simulink model "BoostQuadSimu"  (R2021b)
settings: Solver=VariableStepAuto  StartTime=0.0  StopTime=Tsim  RelTol=1e-3
undefined symbols (not defined in the file): BoostQ, Dc, PRBS_Amp, PRBS_N, PRBS_Ts, Ramp_Max, Tsim
libraries: fl_lib x14, nesl_utility x11, ee_lib x5, spsPWMGeneratorDCDCLib x1
settings Model: Creator=marcus  LastModifiedBy=Gabri
settings SolverCC: AlgebraicLoopSolver=TrustRegion
settings DataIOCC: ReturnWorkspaceOutputs=off
settings DebuggingCC: SFMachineParentedDataDiag=warning  ArithmeticOperatorsInVariantConditions=warning
settings SFSimCC: SimUseLocalCustomCode=off  CustomCodeUndefinedFunction=UseInterfaceOnly
settings RTWCC: RTWUseLocalCustomCode=off

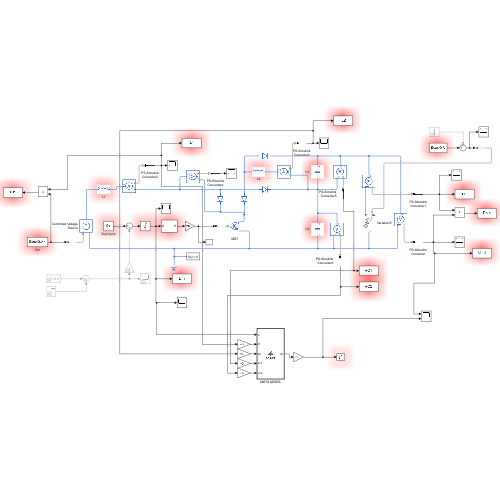
[thumbnail: Simulink's stored preview of the top-level diagram]
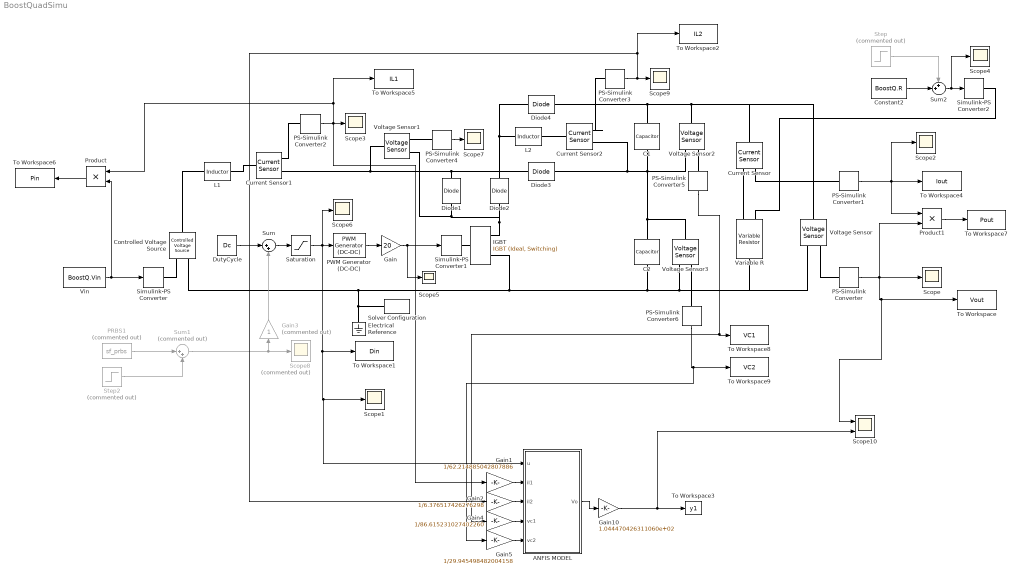
== system BoostQuadSimu ==
  ANFIS MODEL : MATLAB Function  TreatAsAtomicUnit=on
  C1 : fl_lib/Electrical/Electrical Elements/Capacitor  c=BoostQ.C1 F  r=BoostQ.rC1 Ohm  g=0 1/Ohm  i_specify=off  i_priority=None  i=0 A  i_nominal_specify=off  i_nominal_unit=A  i_nominal_value=1  v_specify=on  v_priority=High  v=vc1 V  v_nominal_specify=off  v_nominal_unit=V  v_nominal_value=1  vc_specify=off  vc_priority=None  vc=BoostQ.Vin/2 V  vc_nominal_specify=off  vc_nominal_unit=V  vc_nominal_value=1
  C2 : fl_lib/Electrical/Electrical Elements/Capacitor  c=BoostQ.C2 F  r=BoostQ.rC2 Ohm  g=0 1/Ohm  i_specify=off  i_priority=None  i=0 A  i_nominal_specify=off  i_nominal_unit=A  i_nominal_value=1  v_specify=on  v_priority=High  v=vc2 V  v_nominal_specify=off  v_nominal_unit=V  v_nominal_value=1  vc_specify=off  vc_priority=Low  vc=BoostQ.Vin V  vc_nominal_specify=off  vc_nominal_unit=V  vc_nominal_value=1
  Constant2 : Constant  Value=BoostQ.R
  Controlled Voltage Source : fl_lib/Electrical/Electrical Sources/Controlled Voltage Source
  Current Sensor : fl_lib/Electrical/Electrical Sensors/Current Sensor
  Current Sensor1 : fl_lib/Electrical/Electrical Sensors/Current Sensor
  Current Sensor2 : fl_lib/Electrical/Electrical Sensors/Current Sensor
  Diode{1..4} (4 alike) : ee_lib/Semiconductors & Converters/Diode  ModelType=ee.enum.diode.modelType.pwl  TableType=ee.enum.diode.tableType.IfMat  IfMat=[.07, .12, .19, 1.75, 4.24, 7.32, 11.2; .16, .3, .72, 2.14, 5.02, 8.35, 13.12] A  VfMat=[.9, 1.15, 1.25, 1.5, 1.75, 2.17, 2.6, 2.85; .58, .68, .75, 1.1, 1.38, 1.77, 2.27, 2.7] V  TjVec=[25, 125] degC  VfVec=[.5, .7, .9, 1.3, 1.7, 2.1, 2.5] V  IfVec=[.1, .2, .5, 1, 2, 4, 7, 10] A  Vf=0.01 V  Ron=0.01 Ohm  Goff=1e-5 1/Ohm  prmExp=ee.enum.diode.expParam.useTwo  I12=[.0137, .545] A  V12=[.6, .7] V  RS=0 Ohm  Tmeas=25 degC  IS=1e-12 A  ec=1  I1=0.0137 A  V1=0.6 V  N_series=1  N_parallel=1  Rz=0.3 Ohm  BV=inf V  C_param=ee.enum.diode.capParam.fixed  CJ=0 pF  CJ0=5 pF  Vvec=[.1, 10, 100] V  Cvec=[3.5, 1, .4] pF  VJ=1 V  Mgrad=0.5  FC=0.5  Q_param=ee.enum.diode.recoveryParam.off  iRM=-7.15 A  iF=4 A  didt=-750 A/us  trr_factor=3  trr=115 ns  Qrr=150 nA*s  Vr=-600 V  Ls=150 nH  Erec=0.03 J  TT=50 ns  tau=100 ns  T_param=ee.enum.diode.temperatureParam.off  Tdevice=25 degC  I1_T2=0.245 A  V1_T2=0.5 V  IS_T2=1.25e-7 A  Tmeas2=125 degC  XTI_param=ee.enum.diode.xtiParam.pn  XTI=3  EG_param=ee.enum.diode.egapParam.material_si  EG=1.11 eV  dBVdT=0 V/K  enable_faults=simscape.enum.onoff.off  fault_action=simscape.enum.assert.action.none  fault_types=ee.enum.diode.faults.open  tau_fault=1e-3 s  IfMat_faulted=[.07, .12, .19, 1.75, 4.24, 7.32, 11.2; .16, .3, .72, 2.14, 4.02, 6.35, 9.12] A  VfMat_faulted=[.9, 1.15, 1.25, 1.5, 1.75, 2.17, 2.6, 2.85; .58, .68, .75, 1.1, 1.38, 1.77, 2.27, 2.7] V  VfVec_faulted=[.5, .7, .9, 1.3, 1.7, 2.1, 2.5] V  IfVec_faulted=[.1, .2, .5, 1, 2, 4, 7, 10] A  Ropen_faulted=1000 Ohm  Gshort_faulted=1000 1/Ohm  Vf_faulted=0.6 V  Ron_faulted=0.3 Ohm  Goff_faulted=1e-8 S  I12_faulted=[.0137, .545] A  V12_faulted=[.6, .7] V  IS_faulted=1e-12 A  ec_faulted=1  I1_faulted=0.0137 A  V1_faulted=0.6 V  RS_faulted=0 Ohm  Rz_faulted=0.3 Ohm  BV_faulted=inf V  Cscale_faulted=100  enable_temporal_fault=simscape.enum.onoff.off  t_fault=inf s  enable_behavioral_fault=simscape.enum.onoff.off  max_permissible_voltage=inf V  n_fail_on_voltage=1  max_permissible_current=inf A  t_fail_on_current=1 s  max_permissible_dVdt=inf V/s  i_specify=off  i_priority=None  i=0 A  i_nominal_specify=off  i_nominal_unit=A  i_nominal_value=1  v_specify=off  v_priority=None  v=0 V  v_nominal_specify=off  v_nominal_unit=V  v_nominal_value=1  i_diode_specify=off  i_diode_priority=None  i_diode=0 A  i_diode_nominal_specify=off  i_diode_nominal_unit=A  i_diode_nominal_value=1  v_diode_specify=off  v_diode_priority=None  v_diode=0 V  v_diode_nominal_specify=off  v_diode_nominal_unit=V  v_diode_nominal_value=1  i_capacitor_specify=off  i_capacitor_priority=None  i_capacitor=0 A  i_capacitor_nominal_specify=off  i_capacitor_nominal_unit=A  i_capacitor_nominal_value=1  v_capacitor_specify=off  v_capacitor_priority=None  v_capacitor=0 V  v_capacitor_nominal_specify=off  v_capacitor_nominal_unit=V  v_capacitor_nominal_value=1  power_dissipated_specify=off  power_dissipated_priority=None  power_dissipated=0 W  power_dissipated_nominal_specify=off  power_dissipated_nominal_unit=W  power_dissipated_nominal_value=1  max_permissible_temperature=inf K  t_fail_on_temperature=1 s  thermal_network_parameterization=ee.enum.thermalNetworkTopology.junctionCase  Rth=[0, 10] K/W  Rth_Cauer=[1, 3, 10] K/W  Rth_Foster=[4, 6] K/W  thermal_mass_parameterization=ee.enum.thermalNetwork.timeconstant  thermal_mass=[0, 1] J/K  thermal_mass_Cauer=[.1, .3, 1] J/K  thermal_mass_Foster=[1.5, 3] J/K  thermal_time_constant=[0, 10] s  thermal_time_constant_Cauer=[1, 3, 10] s  thermal_time_constant_Foster=[6, 18] s  thermal_mass_initial_temperatures=[25, 25] degC  thermal_mass_initial_temperatures_Cauer=[25, 25, 25] degC  steadyState_Foster=simscape.enum.onoff.on  Tvec_initial_Foster=[25, 25, 25, 25] degC
  DutyCycle : Constant  Value=Dc
  Electrical Reference : fl_lib/Electrical/Electrical Elements/Electrical Reference
  Gain : Gain  Gain=20
  Gain1 : Gain  Gain=1/62.214885042807886
  Gain10 : Gain  Gain=1.044470426311060e+02
  Gain2 : Gain  Gain=1/6.376517426276298
  Gain3 : Gain  Commented=on
  Gain4 : Gain  Gain=1/86.615231027402260
  Gain5 : Gain  Gain=1/29.945498482004158
  IGBT : ee_lib/Semiconductors & Converters/IGBT (Ideal, Switching)  Vf=0.8 V  Ron=0.001 Ohm  Goff=1e-5 1/Ohm  Vth=6 V  diode_param=1  diode_Vf=0.8 V  diode_Ron=0.001 Ohm  diode_Goff=1e-5 1/Ohm  diode_C=5e-8 F  diode_iRM=-235 A  diode_iF=300 A  diode_idot=-50 A/us  diode_trr_param=1  diode_trr_factor=3  diode_trr=15 us  diode_Qrr=1.5e+3 s*uA  thermal_loss_option=ee.enum.converters.thermalLossOption.constantvalues  Von_data=[0, .1, .6, .8, 1, 1.3, 1.6, 2, 2.4; 0, .1, .7, 1, 1.2, 1.5, 1.9, 2.4, 2.8] V  Tj=[298.15, 398.15] K  Iout_data=[0, .1, 1, 5, 10, 20, 40, 70, 100] A  Eon_data=[0, .0024, .024, .12, .2, .48, 1.04, 2.16, 3.24; 0, .003, .03, .15, .25, .6, 1.3, 2.7, 4.05] * 1e-3 J  Eoff_data=[0, .0007, .0066, .033, .066, .17, .33, .83, 1.5; 0, .001, .01, .05, .1, .25, .5, 1.2, 2.2] * 1e-3 J  Tj_loss=[298.15, 398.15] K  Iout_data_loss=[0, .1, 1, 5, 10, 20, 40, 70, 100] A  Eon_scalar=22.86e-3 J  Eoff_scalar=17.14e-3 J  Voff=300 V  Iout_scalar=600 A  diodeModelType=ee.enum.converters.diodeModelType.pwl  diodeTableType=ee.enum.diode.tableType.IfMat  diode_IfMat=[.07, .12, .19, 1.75, 4.24, 7.32, 11.2; .16, .3, .72, 2.14, 4.02, 6.35, 9.12] A  diode_VfMat=[.9, 1.15, 1.25, 1.5, 1.75, 2.17, 2.6, 2.85; .58, .68, .75, 1.1, 1.38, 1.77, 2.27, 2.7] V  diode_TjVec=[25, 125] degC  diode_VfVec=[.5, .7, .9, 1.3, 1.7, 2.1, 2.5] V  diode_IfVec=[.1, .2, .5, 1, 2, 4, 7, 10] A  diode_Vr=-600 V  diode_Ls=150 nH  diode_Erec=0.03 J  thermal_network_parameterization=ee.enum.thermalNetworkTopology.external  Rth=[.08, .5] K/W  Rth_Cauer=[.08, .1, .5] K/W  Rth_Foster=[.08, .14, .22, .16] K/W  thermal_mass_parameterization=ee.enum.thermalNetwork.timeconstant  thermal_mass=[.01, .5] J/K  thermal_mass_Cauer=[.01, .1, .5] J/K  thermal_mass_Foster=[.001, .005, .05, .5] J/K  thermal_time_constant=[.001, .2] s  thermal_time_constant_Cauer=[.001, .1, .2] s  thermal_time_constant_Foster=[7e-05, .0007, .01, .08] s  thermal_mass_initial_temperatures=[25, 25] degC  thermal_mass_initial_temperatures_Cauer=[25, 25, 25] degC  junction_thermal_mass=0.01 J/K  steadyState_Foster=simscape.enum.onoff.on  Tvec_initial_Foster=[25, 25, 25, 25] degC  no_thermal_network=0  junction_temperature_specify=off  junction_temperature_priority=None  junction_temperature=25 degC  junction_temperature_nominal_specify=off  junction_temperature_nominal_unit=degC  junction_temperature_nominal_value=1  vT_specify=off  vT_priority=None  vT=0 V  vT_nominal_specify=off  vT_nominal_unit=V  vT_nominal_value=1  Qj_specify=off  Qj_priority=None  Qj=0 W  Qj_nominal_specify=off  Qj_nominal_unit=W  Qj_nominal_value=1
  L1 : fl_lib/Electrical/Electrical Elements/Inductor  l=BoostQ.L1 H  r=BoostQ.rL1 Ohm  g=1e-9 1/Ohm  i_specify=on  i_priority=None  i=il1 A  i_nominal_specify=off  i_nominal_unit=A  i_nominal_value=1  v_specify=off  v_priority=None  v=0 V  v_nominal_specify=off  v_nominal_unit=V  v_nominal_value=1  i_L_specify=off  i_L_priority=High  i_L=0 A  i_L_nominal_specify=off  i_L_nominal_unit=A  i_L_nominal_value=1
  L2 : fl_lib/Electrical/Electrical Elements/Inductor  l=BoostQ.L2 H  r=BoostQ.rL2 Ohm  g=1e-9 1/Ohm  i_specify=on  i_priority=None  i=il2 A  i_nominal_specify=off  i_nominal_unit=A  i_nominal_value=1  v_specify=off  v_priority=None  v=0 V  v_nominal_specify=off  v_nominal_unit=V  v_nominal_value=1  i_L_specify=off  i_L_priority=High  i_L=0 A  i_L_nominal_specify=off  i_L_nominal_unit=A  i_L_nominal_value=1
  PRBS1 : S-Function  Commented=on  FunctionName=sf_prbs  Parameters=K,N,Ts  SFunctionDeploymentMode=off  EnableBusSupport=off  mask{K=PRBS_Amp, N=PRBS_N, Ts=PRBS_Ts}
      mask prompts: K "Ganho (K):"; N "Número de Células (usar 5, 7 ou 10):"; Ts "Tempo de amostragem (seg):"
      mask Display: disp('P R B S')
  PS-Simulink Converter{,1..6} (7 alike) : nesl_utility/PS-Simulink Converter  PhysicalDomain=network_engine_domain  SubClassName=ps_output  LeftPortType=input  RightPortType=output  PseudoPeriodic=off  Frequencies=[]  Unit=1  AffineConversion=off
      settings: SourceProductBaseCode=PW,SS
  PWM Generator (DC-DC) : spsPWMGeneratorDCDCLib/PWM Generator (DC-DC)  Fsw=BoostQ.f  Ts=0
  Product : Product
  Product1 : Product
  Saturation : Saturate  UpperLimit=Ramp_Max*1.2  LowerLimit=0
  Scope{,1..7,9} (9 alike) : Scope
  Scope10 : Scope  NumInputPorts=2
  Scope8 : Scope  Commented=on
  Simulink-PS Converter : nesl_utility/Simulink-PS Converter  PhysicalDomain=network_engine_domain  SubClassName=ps_input  LeftPortType=input  RightPortType=output  PseudoPeriodic=off  Frequencies=[]  NoiseDistribution=none  NoiseParameters=[]  Unit=1  AffineConversion=off  FilteringAndDerivatives=provide  SimscapeFilterOrder=1  InputFilterTimeConstant=0.001  UdotUserProvided=0
      settings: SourceProductBaseCode=PW,SS
  Simulink-PS Converter1 : nesl_utility/Simulink-PS Converter  PhysicalDomain=network_engine_domain  SubClassName=ps_input  LeftPortType=input  RightPortType=output  PseudoPeriodic=off  Frequencies=[]  NoiseDistribution=none  NoiseParameters=[]  Unit=1  AffineConversion=off  FilteringAndDerivatives=provide  SimscapeFilterOrder=1  InputFilterTimeConstant=0.001  UdotUserProvided=0
      settings: SourceProductBaseCode=PW,SS
  Simulink-PS Converter2 : nesl_utility/Simulink-PS Converter  PhysicalDomain=network_engine_domain  SubClassName=ps_input  LeftPortType=input  RightPortType=output  PseudoPeriodic=off  Frequencies=[]  NoiseDistribution=none  NoiseParameters=[]  Unit=1  AffineConversion=off  FilteringAndDerivatives=zero  SimscapeFilterOrder=1  InputFilterTimeConstant=0.001  UdotUserProvided=0
      settings: SourceProductBaseCode=PW,SS
  Solver Configuration : nesl_utility/Solver Configuration  PhysicalDomain=network_engine_domain  SubClassName=solver  LeftPortType=input  RightPortType=generic  Tones=[]  Harmonics=[]  SimulateNoise=off  Profile=off  UseLocalSampling=off  EnableSwitchedLinearOptims=on  FrequencyDomain=off  UseCCode=off  RelTol=0.001  AbsTol=1e-06  MinStep=1e-09  ToWorkspace=off  RevertToSquareIcSolve=off  NumHomotopyIterations=100  PhasorMode=off  PhasorModeNumHarmonics=1  DoDC=off  ResidualTolerance=1e-09  UseLocalSolver=off  LocalSolverChoice=NE_BACKWARD_EULER_ADVANCER  LocalSolverSampleTime=0.001  DoFixedCost=off  MaxNonlinIter=3  MaxModeIter=2  ComputeImpulses=off  ImpulseIterations=2  LinearAlgebra=Sparse  EquationFormulation=NE_TIME_EF  DelaysMemoryBudget=1024  AutomaticFiltering=on  FilteringTimeConstant=0.001  PartitionStorageMethod=AS_NEEDED  PartitionMemoryBudget=1024  PartitionMethod=FAST
      settings: SourceProductBaseCode=PW,SS
  Step : Step  Commented=on  Time=Tsim/2  After=-100  SampleTime=0
  Step2 : Step  Commented=on  Time=0  After=0.05  SampleTime=0
  Sum : Sum  Inputs=|++
  Sum1 : Sum  Commented=on  Inputs=|++
  Sum2 : Sum  Inputs=++|
  To Workspace : ToWorkspace  VariableName=Vout  SampleTime=BoostQ.Ts
  To Workspace1 : ToWorkspace  VariableName=Din  SaveFormat=Timeseries  SampleTime=BoostQ.Ts
  To Workspace2 : ToWorkspace  VariableName=IL2  SaveFormat=Timeseries  SampleTime=BoostQ.Ts
  To Workspace3 : ToWorkspace  VariableName=y1  SaveFormat=Timeseries  SampleTime=BoostQ.Ts
  To Workspace4 : ToWorkspace  VariableName=Iout  SaveFormat=Timeseries  SampleTime=BoostQ.Ts
  To Workspace5 : ToWorkspace  VariableName=IL1  SaveFormat=Timeseries  SampleTime=BoostQ.Ts
  To Workspace6 : ToWorkspace  VariableName=Pin  SaveFormat=Timeseries  SampleTime=BoostQ.Ts
  To Workspace7 : ToWorkspace  VariableName=Pout  SaveFormat=Timeseries  SampleTime=BoostQ.Ts
  To Workspace8 : ToWorkspace  VariableName=VC1  SaveFormat=Timeseries  SampleTime=BoostQ.Ts
  To Workspace9 : ToWorkspace  VariableName=VC2  SaveFormat=Timeseries  SampleTime=BoostQ.Ts
  Variable R : fl_lib/Electrical/Electrical Elements/Variable Resistor  Rmin=0 Ohm  i_specify=off  i_priority=None  i=0 A  i_nominal_specify=off  i_nominal_unit=A  i_nominal_value=1  v_specify=off  v_priority=None  v=0 V  v_nominal_specify=off  v_nominal_unit=V  v_nominal_value=1
  Vin : Constant  Value=BoostQ.Vin
  Voltage Sensor{,1..3} (4 alike) : fl_lib/Electrical/Electrical Sensors/Voltage Sensor
  wires:
  Vin/1 -> Simulink-PS Converter/1, Product/2
  PWM Generator (DC-DC)/1 -> Gain/1
  Constant2/1 -> Sum2/2
  Step/1 -> Sum2/1
  PS-Simulink Converter1/1 -> Product1/1, Scope2/1, To Workspace4/1
  PS-Simulink Converter2/1 -> Gain1/1, Product/1, To Workspace5/1, Scope3/1
  Sum2/1 -> Scope4/1, Simulink-PS Converter2/1
  Product/1 -> To Workspace6/1
  Product1/1 -> To Workspace7/1
  PS-Simulink Converter4/1 -> Scope7/1
  DutyCycle/1 -> Sum/1
  PRBS1/1 -> Sum1/1
  Gain/1 -> Simulink-PS Converter1/1, Scope5/1
  PS-Simulink Converter/1 -> Scope10/1, To Workspace/1, Product1/2, Scope/1
  Step2/1 -> Sum1/2
  Sum1/1 -> Gain3/1, Scope8/1
  Gain3/1 -> Sum/2
  Sum/1 -> Saturation/1
  PS-Simulink Converter3/1 -> Gain2/1, To Workspace2/1, Scope9/1
  PS-Simulink Converter6/1 -> Gain5/1, To Workspace9/1
  PS-Simulink Converter5/1 -> Gain4/1, To Workspace8/1
  ANFIS MODEL/1(Vo) -> Gain10/1
  Gain10/1 -> Scope10/2, To Workspace3/1
  Saturation/1 -> Scope6/1, PWM Generator (DC-DC)/1, ANFIS MODEL/1(u), Scope1/1, To Workspace1/1
  Gain1/1 -> ANFIS MODEL/2(il1)
  Gain2/1 -> ANFIS MODEL/3(il2)
  Gain4/1 -> ANFIS MODEL/4(vc1)
  Gain5/1 -> ANFIS MODEL/5(vc2)
  connections:
  L1/LConn1 -- Controlled Voltage Source/LConn1
  Simulink-PS Converter/RConn1 -- Controlled Voltage Source/RConn1
  Controlled Voltage Source/RConn2 -- IGBT/RConn2 -- Voltage Sensor3/RConn2 -- Voltage Sensor/RConn2 -- Variable R/RConn1 -- C2/RConn1 -- Solver Configuration/RConn1 -- Electrical Reference/LConn1
  IGBT/LConn1 -- Simulink-PS Converter1/RConn1
  Current Sensor1/RConn2 -- Voltage Sensor1/LConn1 -- Diode1/LConn1 -- Diode3/LConn1
  Diode1/RConn1 -- Voltage Sensor1/RConn2 -- Diode2/RConn1 -- IGBT/RConn1
  Simulink-PS Converter2/RConn1 -- Variable R/LConn1
  Diode3/RConn1 -- Current Sensor2/RConn2 -- Voltage Sensor2/RConn2 -- C1/RConn1 -- Voltage Sensor3/LConn1 -- C2/LConn1
  Diode4/RConn1 -- Voltage Sensor2/LConn1 -- Current Sensor/LConn1 -- Voltage Sensor/LConn1 -- C1/LConn1
  Diode4/LConn1 -- Diode2/LConn1 -- L2/LConn1
  Voltage Sensor/RConn1 -- PS-Simulink Converter/LConn1
  Current Sensor/RConn2 -- Variable R/LConn2
  PS-Simulink Converter1/LConn1 -- Current Sensor/RConn1
  Current Sensor1/LConn1 -- L1/RConn1
  PS-Simulink Converter2/LConn1 -- Current Sensor1/RConn1
  PS-Simulink Converter4/LConn1 -- Voltage Sensor1/RConn1
  Current Sensor2/LConn1 -- L2/RConn1
  Current Sensor2/RConn1 -- PS-Simulink Converter3/LConn1
  PS-Simulink Converter5/LConn1 -- Voltage Sensor2/RConn1
  Voltage Sensor3/RConn1 -- PS-Simulink Converter6/LConn1

== matlab function BoostQuadSimu/ANFIS MODEL ==
  settings: updateMethod=DISCRETE  sampleTime=BoostQ.Ts
  data: u input; Vo output; il1 input; il2 input; vc1 input; vc2 input
function Vo = ANFIS(u, il1, il2, vc1, vc2)
persistent b1 mean1 sigma1 ThetaL4 Mi NumInVars NumInTerms NumRules uo vo 

if isempty(Mi)
    uo = u;
    vo = 30/1.044470426311060e+02;
    Mi          = 7;
    NumInVars   = Mi;
    NumInTerms  = 7;
    NumRules = NumInTerms;
    
    b1 = [-44.0573249198801,-3.01318228051362,-13.6834056692177,5.39229512944622,8.65943640411405,5.43090099217590,-11.7574885245845;-34.3161545180684,110.735628861312,3.07245327629263,-33.0859943643098,-8.81749579181387,-128.488946681374,22.4316392854820;-123.108169235995,3.34528448319628,-14.7383081893959,15.7335876926653,10.1801527697701,65.9173989576329,-34.7500391619463;-6.70405982410581,-29.6048184503747,-21.3043228534210,-8.56967092616348,-14.4044713928412,52.0065608219453,63.5990220338469;22.8005873682614,10.4961534227908,-14.5037878890356,10.3376165350608,-4.80421733066544,-49.1136959446346,-137.006217332172;69.0794273784091,7.20203931365437,-19.0034235694986,7.62958843330971,-10.2178561921036,16.1178375209470,4.41059662976930;-65.4743326214945,47.3618856245921,-27.5599232595838,0.941389117178850,-11.5505637695882,-13.7922811626365,-263.606950367280]; 
    mean1 = [-353.558410197683,-38.8880222148552,5.40142914619578,6.80853915779209,9.48449270370711,20.2424691642285,34.2647687468822;-222.225262763012,-36.7798595978532,3.94923031601152,8.66615507724804,32.6731414958159,93.7841352029563,502.990966979516;-168.273615611018,-0.399546403788738,24.8213308495999,27.6770070878262,30.1875214694559,45.2307556648521,124.641408677142;3.41273273593276,11.1765159683727,21.5977530907096,26.1026649090919,29.3642358964460,36.8977650733427,111.063342031655;-13.5966405704134,4.15076976320543,5.51669315268063,6.59974296281747,20.3392757558742,63.6275550199403,1217.87059690949;-46.4150986304193,-14.1696201346101,0.374268520037133,10.7766774391450,33.4573043016600,74.9419370136020,95.6169180136497;-123.600518262858,-19.9535936636326,-6.90175211385527,2.49199762884177,4.75861316945817,8.93053730527283,405.541790177747];
    sigma1 = [-232.089887129330,81.2571209681163,4.53961203966865,-3.84929711760597,5.50035084162194,-15.1702256916638,-14.1113843532041;150.397662050080,176.656320508728,1.08286037884481,3.18378146988815,47.1906102979283,120.635680227603,-8.11517844311309;-80.9139823674148,-8.59199912614853,48.4233928427262,4.63210725410515,-37.5392641668837,-81.6468481741995,51.7976055278881;-1.55017614734290,65.4472334927356,18.3353485688629,8.87180573961267,-12.6148857235093,66.0053247804628,80.7361205456110;36.6025944971823,14.2740916422147,3.89839744610439,10.7401486787670,6.85239853705069,27.5763031280418,109.089420798546;91.1749243364195,24.2483774104017,-30.8412690351411,-4.63599182139312,21.7248364778519,-88.4261250755028,-34.1716571821792;19.5193979090080,-94.0672107010295,-5.32139343457962,0.971146841504750,7.01543226090493,-13.0271777374607,171.284302806004];
    ThetaL4 = [-0.153555572809097;0.149746915930402;0.410621015454787;-0.0129790885509411;-0.0196556638796432;0.487412969953205;0.170476444169948;-0.00190356205581022;5814.63551577469;5814.77854667134;-36574.6337839047;-146262.662472782;35697.0539481796;-195036.751813150;436562.236910930;-424366.148134832;-19043.2582750946;-19043.1166400735;78824.0382060923;10572.4701027861;-115124.981889694;55640.4858281335;113997.196968512;-165606.417692860;-62442.3675632557;-62442.3489457048;-37872.3617710610;42711.0311518595;-346089.702802060;-20368.5553197567;-73178.2422722943;96116.6410661992;-52010.5743668421;-52011.0005567096;23034.1074440663;44915.9111243212;-370206.668828496;3569.32188381144;70016.7787876976;119330.251234137;188956.038150015;188955.796528095;-77573.9535202018;84401.9464049275;-685456.909928298;-10468.2582348613;-240290.639127713;-58134.8468008718;-91201.8288621800;-91201.9885440665;-31748.2338626064;1143.20159346931;-11956.7876970884;5170.18012366402;-125687.999656450;-150849.596538010]; 
    Vo = vo;
    return
end
In1 = [uo; u; vo; il1; il2; vc1; vc2];

% LAYER 1 - INPUT TERM NODES
In2 = In1*ones(1,NumInTerms);
Out1 = 1./(1 + (abs((In2-mean1)./sigma1)).^(2*b1));

% LAYER 2 - PRODUCT NODES
Out2 = prod(Out1,1);
S_2 = sum(Out2);

% LAYER 3 - NORMALIZATION NODES
if S_2~=0
    Out3 = Out2'/S_2;
else
    Out3 = zeros(1,NumRules);
end

% LAYERS 4 - 5: CONSEQUENT NODES - SUMMING NODE
Aux1 = [In1; 1]*Out3';

% New Input Training Data shaped as a column vector.
a = reshape(Aux1,(NumInVars+1)*NumRules,1);

vo_a = a'*ThetaL4;

vo = vo_a;
uo = u;

Vo = vo_a;
